simulink model "TestbenchSubsystem"  (R2019b)
settings: Solver=VariableStepAuto  StartTime=0.0  StopTime=10.0  RelTol=1e-3
values from neighbouring files (symbols this model uses):
  bo = b0/(c*a1)    [otpADRC.m]
  wc = 1/(c*a1)    [otpADRC.m]
undefined symbols (not defined in the file or in its folder): A, B, C, D, obs
libraries: simulink x1
settings Model: Creator=didi  LastModifiedBy=didi

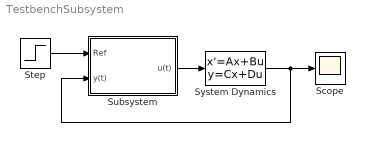
== system TestbenchSubsystem ==
  Scope : Scope
  Step : Step  SampleTime=0
  Subsystem : Subsystem
  System Dynamics : StateSpace  A=A  B=B  C=C  D=D  InitialCondition=0
  wires:
  Step/1 -> Subsystem/1(Ref)
  System Dynamics/1 -> Subsystem/2(y(t)), Scope/1
  Subsystem/1(u(t)) -> System Dynamics/1

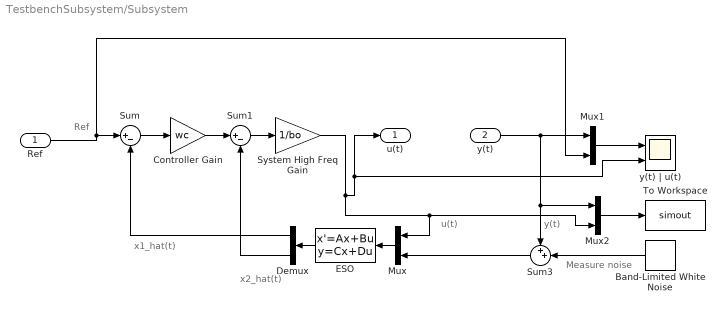
== system TestbenchSubsystem/Subsystem ==
  note: y(t)
  note: x2_hat(t)
  note: Measure noise
  note: Ref
  note: u(t)
  note: x1_hat(t)
  Ref : Inport
  y(t) : Inport  Port=2
  Band-Limited White Noise : simulink/Sources/Band-Limited White Noise  Cov=[0.000001]  Ts=0.76  seed=[23341]
  Controller Gain : Gain  Gain=wc
  Demux : Demux  Outputs=2
  ESO : StateSpace  A=obs.A  B=obs.B  C=obs.C  D=obs.D  InitialCondition=0
  Mux : Mux  Inputs=2
  Mux1 : Mux  Inputs=2
  Mux2 : Mux  Inputs=2
  Sum : Sum  Inputs=|+-
  Sum1 : Sum  Inputs=|+-
  Sum3 : Sum  Inputs=++|
  System High Freq Gain : Gain  Gain=1/bo
  To Workspace : ToWorkspace  VariableName=simout  SaveFormat=Timeseries  SampleTime=-1
  y(t) | u(t) : Scope  NumInputPorts=2
  u(t) : Outport
  wires:
  Mux2/1 -> To Workspace/1
  Band-Limited White Noise/1 -> Sum3/2
  Sum1/1 -> System High Freq Gain/1
  Demux/1 -> Sum/2
  Ref/1 -> Mux1/2, Sum/1
  Sum3/1 -> Mux/2
  Mux1/1 -> y(t) | u(t)/1
  ESO/1 -> Demux/1
  y(t)/1 -> Mux2/1, Sum3/1, Mux1/1
  Sum/1 -> Controller Gain/1
  Controller Gain/1 -> Sum1/1
  Mux/1 -> ESO/1
  Demux/2 -> Sum1/2
  System High Freq Gain/1 -> Mux2/2, Mux/1, u(t)/1, y(t) | u(t)/2
